simulink model "control_block"  (R2025b)
settings: Solver=FixedStepDiscrete  StartTime=0.0  StopTime=5  FixedStep=1e-4  RelTol=1e-3
model workspace (MAT data in the model file):
  Ki_speed : Simulink.Parameter (value not decoded)
  Kp_speed : Simulink.Parameter (value not decoded)
undefined symbols (not defined in the file): airgap_vec, angulos, DiscIntNeverNeededParam, Distance_between_EMS, force_drag_vec, frac_polar, fuerza, hems_n, init_angle_from_speetec, initial_angle, initial_speed, kd, magnitude, mass, max_voltage, real_airgap, Resistencia, speed_drag_vec, speed_reference_ms, speetec_end, speetec_init, speetec_offset
libraries: slpidlib x2, simulink x1
(part 2 of 2)

== matlab function control_block/PLANT/LSM model/Maximun calculation/Frequency and Max Calculator ==
  settings: updateMethod=DISCRETE  sampleTime=1e-4
  data: frecuencia output; value input; Maximo output
function [frecuencia,Maximo]= fcn(value)

%#codegen

% Calculate Frequency and max peak

Ts = 1e-4;

persistent tiempo
if isempty(tiempo)
    tiempo = 0;
end

tiempo = tiempo + Ts;

frecuencia = frecuency_calculator(value, tiempo);
Maximo = maximum_calculator(frecuencia, value, tiempo);

end


% ============================================================
% Calculate Frequency
% ============================================================

function frecuencia = frecuency_calculator(value, tiempo)

persistent signo
if isempty(signo)
   signo = [0 0 0];
end

persistent t_inicio
if isempty(t_inicio)
   t_inicio = [0 0 0];
end

persistent frecuencia_acc
if isempty(frecuencia_acc)
   frecuencia_acc = 1;
end

frecuencia = frecuencia_acc;

for i = 1:3

    if signo(i) == 0

        if value(i) >= 0
            signo(i) = 1;
        else
            signo(i) = 2;
        end

        t_inicio(i) = tiempo;

    end

    if signo(i) == 1

        if value(i) <= 0

            dt = tiempo - t_inicio(i);

            % avoid division by zero
            if dt > 1e-12

                frecuencia = 1 / (2 * dt);
                frecuencia_acc = frecuencia;

            end

            signo(i) = 0;

        end

    end

    if signo(i) == 2

        if value(i) >= 0

            dt = tiempo - t_inicio(i);

            % avoid division by zero
            if dt > 1e-12

                frecuencia = 1 / (2 * dt);
                frecuencia_acc = frecuencia;

            end

            signo(i) = 0;

        end

    end

end

end


% ============================================================
% Calculate Max value
% ============================================================

function Maximo = maximum_calculator(frecuencia, valor, tiempo)

persistent antiguo_maximo
if isempty(antiguo_maximo)
   antiguo_maximo = 0;
end

persistent t_maximo
if isempty(t_maximo)
   t_maximo = 0;
end

maximo = [0 0 0];

frecuencia_abs = abs(frecuencia);

% avoid division by zero
if frecuencia_abs < 1e-12
    frecuencia_abs = 1e-12;
end

periodo = 1 / frecuencia_abs / 3;

for i = 1:3

    if abs(valor(i)) >= antiguo_maximo

        maximo(i) = abs(valor(i));
        antiguo_maximo = abs(valor(i));
        t_maximo = tiempo;

    else

        maximo(i) = antiguo_maximo;

        if tiempo > t_maximo + periodo

            maximo(i) = abs(valor(i));
            antiguo_maximo = abs(valor(i));
            t_maximo = tiempo;

        end

    end

end

Maximo = max(maximo);

end

% function [frecuencia,Maximo]= fcn(value)
%  % Calculate Frequency and max peak
%  Ts = 1e-4;
% 
% persistent tiempo
% if isempty(tiempo)
%     tiempo = 0;
% end
% 
% tiempo = tiempo + Ts;
% 
% frecuencia = frecuency_calculator(value, tiempo);
% Maximo = maximum_calculator(frecuencia, value, tiempo);
% 
% end
% 
% % Calculate Frequency
% function frecuencia = frecuency_calculator(value, tiempo)
%     persistent signo
%     if isempty(signo)
%        signo = [0 0 0]; 
%     end
%     persistent t_inicio
%     if isempty(t_inicio)
%        t_inicio = [0 0 0];
%     end
%     persistent frecuencia_acc
%     if isempty(frecuencia_acc)
%        frecuencia_acc = 1;
%     end
% 
%     frecuencia = frecuencia_acc;
%     for i = 1:3
%         if signo(i) == 0
%             if value(i) >= 0 
%                 signo(i) = 1;
%             else
%                 signo(i) = 2;
%             end
%             t_inicio(i) = tiempo;
%         end
% 
%         if signo(i) == 1
%             if value(i) <= 0
%                 frecuencia = 1 / (2 * (tiempo - t_inicio(i)));
%                 frecuencia_acc = frecuencia;
%                 signo(i) = 0;
%             end
%         end
% 
%         if signo(i) == 2
%             if value(i) >= 0
%                 frecuencia = 1 / (2 * (tiempo - t_inicio(i)));
%                 frecuencia_acc = frecuencia;
%                 signo(i) = 0;
%             end
%         end
%     end
% end
% % Calculate Max value
% function Maximo = maximum_calculator(frecuencia, valor, tiempo)
%     persistent antiguo_maximo
%     if isempty(antiguo_maximo)
%        antiguo_maximo = 0;
%     end
%     persistent t_maximo
%     if isempty(t_maximo)
%        t_maximo = 0;
%     end
% 
%     maximo = [0 0 0];
%     periodo = 1 / abs(frecuencia) / 3;
%     for i = 1:3
%         if abs(valor(i)) >= antiguo_maximo
%             maximo(i) = abs(valor(i));
%             antiguo_maximo = abs(valor(i));
%             t_maximo = tiempo;
%         else
%             maximo(i) = antiguo_maximo;
%             if tiempo > t_maximo + periodo
%                 maximo(i) = abs(valor(i));
%                 antiguo_maximo = abs(valor(i));
%                 t_maximo = tiempo;
%             end
%         end
%     end
%     Maximo = max(maximo);
% end

== matlab function control_block/PLANT/LSM model/Sensor de Corriente/Sensor corriente U/Sensor ==
  data: I input; V output; Offset input
function V = fcn(I, Offset)

Vcc = 5;                                        %Vcc ??                             La corriente va hasta máximo 5V

if (I > 300)
    I = 300;
end

if (I < -300)
    I = -300;
end


V_ref = Vcc / 2;

V = V_ref + 0.005 * I;

V = V + Offset;                 % Por?


end

== matlab function control_block/PLANT/LSM model/Sensor de Corriente/Sensor corriente U/Discretizado Amplitud ==
  data: valor input; valor_discretizado output; num_valores input; max input; min input
function valor_discretizado = fcn(valor, num_valores, max, min)

if valor > max
    valor_discretizado = max;
    return
end

if valor < min
    valor_discretizado = min;
    return
end


valor_escalon = (max - min)/(num_valores - 1);


i = min;


while (i < max)
    if (i + valor_escalon/2 > valor)
        valor_discretizado = i;
        return
    end

    i = i + valor_escalon;
end


valor_discretizado = max;

end

== matlab function control_block/PLANT/LSM model/Sensor de Corriente/Sensor corriente U/MATLAB Function1 ==
  data: V input; I output
function I = fcn(V)

I = (V - 2.5)/0.005;

== matlab function control_block/PLANT/LSM model/Sensor de Corriente/Sensor corriente V/Discretizado Amplitud ==
  data: valor input; valor_discretizado output; num_valores input; max input; min input
function valor_discretizado = fcn(valor, num_valores, max, min)

if valor > max
    valor_discretizado = max;
    return
end

if valor < min
    valor_discretizado = min;
    return
end


valor_escalon = (max - min)/(num_valores - 1);


i = min;


while (i < max)
    if (i + valor_escalon/2 > valor)
        valor_discretizado = i;
        return
    end

    i = i + valor_escalon;
end


valor_discretizado = max;

end

== matlab function control_block/PLANT/LSM model/Sensor de Corriente/Sensor corriente V/MATLAB Function1 ==
  data: V input; I output
function I = fcn(V)

I = (V - 2.5)/0.005;

== matlab function control_block/PLANT/LSM model/Sensor de Corriente/Sensor corriente V/Sensor ==
  data: I input; V output; Offset input
function V = fcn(I, Offset)

Vcc = 5;                                        %Vcc ??                             La corriente va hasta máximo 5V

if (I > 300)
    I = 300;
end

if (I < -300)
    I = -300;
end


V_ref = Vcc / 2;

V = V_ref + 0.005 * I;

V = V + Offset;                 % Por?


end
